simulink model "dvbs2hdlTransmitterCore"  (R2024b)
settings: Solver=FixedStepDiscrete  StartTime=0.0  StopTime=0  RelTol=1e-3
libraries: hdlsllib x105, simulink x41, dspsigops x7, commseqgen3 x5, whdlutilities x5, commhdlcrc x2, dsphdlfiltering2 x1, whdlmod x1
(part 5 of 5)

== system dvbs2hdlTransmitterCore/DVB-S2 Tx/Interleaver/DVB-S2 HDL Interleaver/RAM Address Generator/Read Offset Address/Read Offset Address Signals Generator/FIFO 3 Variables/No HDL/No HDL ==
  wr : Inport
  full : Inport  Port=2
  ncount : Inport  Port=3
  empty : Inport  Port=4
  rd : Inport  Port=5
  Assertion : Assertion  AssertionFailFcn=warning('push on to a full RAM');  StopWhenAssertionFail=off
  Assertion1 : Assertion  AssertionFailFcn=warning('pop from an empty RAM');  StopWhenAssertionFail=off
  Display : Display
  Logical Operator : Logic  Operator=NAND  AllPortsSameDT=off  OutDataTypeStr=boolean
  Logical Operator1 : Logic  Operator=NAND  AllPortsSameDT=off  OutDataTypeStr=boolean
  wires:
  rd/1 -> Logical Operator1/2
  Logical Operator/1 -> Assertion/1
  empty/1 -> Logical Operator1/1
  ncount/1 -> Display/1
  full/1 -> Logical Operator/2
  wr/1 -> Logical Operator/1
  Logical Operator1/1 -> Assertion1/1

== matlab function dvbs2hdlTransmitterCore/DVB-S2 Tx/FEC Encoder/DVB-S2 BCH Encoder/Input controller/Sample Frame type and code rate ==
  data: Enable input; inpFrameLength output; frameTypeIn input; codeRateIdxIn input; inpParityLength output; validateFrameFlag output
function [inpFrameLength,inpParityLength,validateFrameFlag] = sampFramTypeCodeRate(Enable,frameTypeIn,codeRateIdxIn)
%#codegen
%% LUT
inputNFramLenLUT = fi([16008 21408 25728 32208 38688 43040 48408 51648 53840 57472 58192 58192 58192 58192 58192 58192]-1,0,16,0);
inputSFramLenLUT = fi([ 3072  5232  6312  7032  9552 10632 11712 12432 13152 14232 14232 14232 14232 14232 14232 14232]-1,0,14,0);

inpParityNLenLUT = fi([192 192 192 192 192 160 192 192 160 128 128 128 128 128 128 128 ]-1,0,8,0);
inpParitySLenLUT = fi([168 168 168 168 168 168 168 168 168 168 168 168 168 168 168 168]-1,0,8,0);
validateFrameLUT = fi([0 1],0,1,0);

inpFrameLength=cast(0,'like',inputNFramLenLUT);
inpParityLength = cast(0,'like',inpParityNLenLUT);
validateFrameFlag = cast(0,'like',validateFrameLUT);

persistent frameLength;
if isempty(frameLength)
    frameLength=cast(0,'like',inputNFramLenLUT);
end

persistent parityLength;
if isempty(parityLength)
    parityLength=cast(0,'like',inpParityNLenLUT);
end

persistent validateFrame;
if isempty(validateFrame)
    validateFrame=cast(0,'like',validateFrameLUT);
end

%% fetch from inputFramLenLUT
if Enable
    if (~frameTypeIn && codeRateIdxIn <= 10 ) || ( frameTypeIn && codeRateIdxIn <= 9 )
        validateFrameFlag(:) = validateFrameLUT(2);
        validateFrame(:) = validateFrameFlag;
    else
        validateFrameFlag(:) = validateFrameLUT(1);
        validateFrame(:) = validateFrameFlag;
    end
    if frameTypeIn
        inpFrameLength(:)=inputSFramLenLUT(codeRateIdxIn+1);
        frameLength(:)=inputSFramLenLUT(codeRateIdxIn+1);
        inpParityLength(:)=inpParitySLenLUT(codeRateIdxIn+1);
        parityLength(:)=inpParitySLenLUT(codeRateIdxIn+1);
    else
        inpFrameLength(:)=inputNFramLenLUT(codeRateIdxIn+1);
        frameLength(:)=inputNFramLenLUT(codeRateIdxIn+1);
        inpParityLength(:)=inpParityNLenLUT(codeRateIdxIn+1);
        parityLength(:)=inpParityNLenLUT(codeRateIdxIn+1);
    end
else
    inpFrameLength(:)=frameLength;
    inpParityLength(:)=parityLength;
    validateFrameFlag(:) = validateFrame;
end
end

== matlab function dvbs2hdlTransmitterCore/DVB-S2 Tx/FEC Encoder/DVB-S2 BCH Encoder/Input controller/sample bus controller function ==
  data: startIn input; sampledStartIn output; endIn input; validIn input; sampledEndIn output; enbBCHEnc output; reset output
function [sampledStartIn,sampledEndIn,enbBCHEnc,reset] = sampleBusController(startIn,endIn,validIn)
%#codegen
persistent startInTempFlag;
persistent endInFlag;

if isempty(startInTempFlag)
    startInTempFlag =  fi(0,0,1,0);
end
if isempty(endInFlag)
    endInFlag =  fi(0,0,1,0);
end

if endInFlag==1
    startInTempFlag = fi(0,0,1,0);
    endInFlag = fi(0,0,1,0);
end

if startIn==1 && validIn==1 && endIn~=1
    if startInTempFlag==1
        reset = fi(1,0,1,0); %reset
    else
        reset = fi(0,0,1,0);
    end
    sampledStartIn = fi(1,0,1,0); %startSample
    startInTempFlag = fi(1,0,1,0);
else
    sampledStartIn = fi(0,0,1,0);
    reset = fi(0,0,1,0);
end

if startInTempFlag
    enbBCHEnc = fi(1,0,1,0);
else
    enbBCHEnc = fi(0,0,1,0); 
end

if startIn~=1 && endIn==1 && validIn==1 && endInFlag~=1 && startInTempFlag==1
    sampledEndIn = fi(1,0,1,0);
    endInFlag = sampledEndIn;
else
    sampledEndIn = fi(0,0,1,0);
end

== matlab function dvbs2hdlTransmitterCore/DVB-S2 Tx/FEC Encoder/DVB-S2 BCH Encoder/Parity Generation/parity indexing ==
  data: parityVectorInp input; parityScalarOut output; parityScalarValid input; parityIndex input; parityScalarValidOut output; parityLength input
function [parityScalarOut,parityScalarValidOut] = parityIndexing(parityVectorInp,parityScalarValid,parityIndex,parityLength)
%#codegen

parityScalarOut = cast(zeros(1,1),'like',parityScalarValid);
parityScalarValidOut = cast(zeros(1,1),'like',parityScalarValid);

if parityScalarValid 
    parityScalarOut(:) = parityVectorInp(parityIndex+1);
    parityScalarValidOut(:) = parityScalarValid;
else
    parityScalarOut(:) = zeros(1,1);
    parityScalarValidOut(:) = zeros(1,1);
end

== matlab function dvbs2hdlTransmitterCore/DVB-S2 Tx/FEC Encoder/DVB-S2 BCH Encoder/Parity Generation/update parity bits ==
  data: readInpData input; parityBitsVector output size=192; readInpValid input; ParityCalCompFlag input; parityValidVector output; parityValid output; parityLength input; reset input
function [parityBitsVector,parityValidVector,parityValid] = parityBitsUpdater(readInpData,readInpValid,ParityCalCompFlag,parityLength,reset)
%#codegen

persistent writeParData;

parityBuffLen = 192;

if isempty(writeParData) || reset
    writeParData = cast(zeros(parityBuffLen,1),'like',readInpData);
end

parityBits =  cast(zeros(parityBuffLen,1),'like',readInpData);
parityBits(:) =  writeParData;
parityBitsVector = cast(zeros(parityBuffLen,1),'like',readInpData);
parityValidVector = cast(zeros(parityBuffLen,1),'like',readInpData);
parityValid = cast(zeros(1,1),'like',readInpData);
genPoly = cast(zeros(193,1),'like',readInpData);

genPoly192 = cast([1  1   1  0  0  1  1  1  1  0  1  0  1  0  1  0  0  1  0 ...
    0  0  0  0  0  0  1  1  0  0  1  1  0  1  1  1  0  1  1 ...
    1  1  1  0  1  0  0  0  0  1  1  1  1  0  0  0  1  0  1 ...
    1  0  0  0  0  0  0  1  0  0  1  0  0  0  1  0  0  0  1 ...
    0  0  0  0  1  0  1  0  1  1  0  0  0  0  1  1  1  0  1 ...
    1  0  0  0  1  1  0  1  1  0  0  1  1  0  1  0  0  1  1 ...
    1  1  0  0  1  1  0  0  0  0  1  0  1  0  0  0  1  1  1 ...
    0  0  0  1  0  0  0  1  0  1  0  0  0  1  1  1  0  1  0 ...
    0  0  1  0  0  0  0  1  1  1  0  0  0  0  0  1  0  1  1 ...
    1  0  0  0  0  0  1  1  0  0  1  0  0  0  1  1  1  0  0 ...
    1  0  1]','like',readInpData);
genPoly168 = cast([1  0  1  0  0  1  0  1  1  0  1  0  0  0  0  0  1  0  0 ...
    1  1  0  0  0  1  0  0  0  1  0  1  1  1  1  1  0  1  0 ...
    1  1  1  1  1  0  0  1  1  1  1  1  1  1  0  0  0  1  0 ...
    1  0  0  1  0  1  0  1  0  0  1  0  1  1  0  0  0  0  0 ...
    1  0  0  1  1  1  0  0  0  1  0  1  1  1  0  0  0  1  0 ...
    0  1  0  1  1  0  0  1  1  0  1  0  0  0  1  1  0  0  1 ...
    0  0  1  1  0  1  1  0  0  1  0  1  1  0  0  0  0  1  1 ...
    0  0  1  0  1  0  1  0  1  1  1  1  1  0  1  1  0  1  1 ...
    0  1  0  0  0  1  1  0  0  0  0  0  0  0  1  0  1]','like',readInpData);
genPoly160 = cast([1  0  0  0  1  0  0  1  1  0  1  0  0  1  1  0  1  1  0 ...
    1  1  1  0  1  0  0  0  1  1  1  0  1  1  0  0  0  0  0 ...
    0  0  1  1  0  0  0  1  0  0  1  0  0  0  1  0  1  1  1 ...
    1  1  1  0  1  1  1  1  1  0  0  0  0  0  0  1  1  1  0 ...
    1  0  1  0  0  0  0  1  1  1  1  0  0  1  0  1  0  1  1 ...
    0  1  1  1  1  1  0  0  0  1  1  0  0  1  1  0  0  0  1 ...
    0  1  0  1  0  0  0  0  1  1  1  1  1  1  1  0  1  1  0 ...
    1  1  1  0  0  1  1  0  0  0  0  1  0  1  0  1  0  0  0 ...
    0  0  0  0  0  1  1  0  1]','like',readInpData);
genPoly128 = cast([1  1  0  1  0  1  0  0  0  1  1  0  0  1  1  0  1  0  0 ...
    1  1  1  1  1  0  0  1  0  0  0  0  0  1  0  1  0  1  1 ...
    1  0  1  0  1  1  0  1  1  0  0  0  1  1  1  1  1  1  1 ...
    0  0  1  1  0  0  0  1  0  1  1  1  1  0  1  1  1  1  0 ...
    1  0  0  1  1  1  1  0  0  1  0  0  1  0  0  0  1  1  1 ...
    0  1  1  1  1  1  0  1  0  1  0  1  0  0  1  0  0  1  1 ...
    1  0  0  0  0  0  0  0  1  1  1  0  0  0  1]','like',readInpData);
switch parityLength
    case 191
        genPoly(:) = genPoly192;
    case 167
        genPoly(:) = [false(192-168,1); genPoly168 ];
    case 159
        genPoly(:) = [false(192-160,1); genPoly160 ];
    case 127
        genPoly(:) = [false(192-128,1); genPoly128 ];
    otherwise
        genPoly(:) = false(193,1);
end
parityLen192 = length(genPoly192)-1;
if readInpValid
    d = xor(readInpData, parityBits(192));
    for idxPoly = parityLen192 : -1 : 2
        if idxPoly > 192-parityLength
            parityBits(idxPoly) = xor(parityBits(idxPoly-1), (genPoly(idxPoly) & d));
        else
            parityBits(idxPoly) = false;
        end
    end
    parityBits(192-parityLength) = d;
    writeParData(:) = parityBits;
else
    parityBits(:) = writeParData;
end

if ParityCalCompFlag && parityLength == 191
    parityBitsVector(:) = flip(parityBits);
    parityValidVector(:) = ones(parityBuffLen,1);
    parityValid(:) = ones(1,1);
elseif ParityCalCompFlag && parityLength == 167
    parityBitsVector(:) = [flip(parityBits((192-167):192)); false(192-168,1)];
    parityValidVector(:) = [ones(168,1) ; zeros(192-168,1)];
    parityValid(:) = ones(1,1);
elseif ParityCalCompFlag && parityLength == 159
    parityBitsVector(:) = [flip(parityBits((192-159):192)); false(192-160,1)];
    parityValidVector(:) = [ones(160,1) ; zeros(192-160,1)];
    parityValid(:) = ones(1,1);
elseif ParityCalCompFlag && parityLength == 127
    parityBitsVector(:) = [flip(parityBits((192-127):192)); false(192-128,1)];
    parityValidVector(:) = [ones(128,1) ; zeros(192-128,1)];
    parityValid(:) = ones(1,1);
else
    parityBitsVector(:) = zeros(parityBuffLen,1);
    parityValidVector(:) = zeros(parityBuffLen,1);
    parityValid(:) = zeros(1,1);
end

== matlab function dvbs2hdlTransmitterCore/DVB-S2 Tx/FEC Encoder/DVB-S2 LDPC Encoder/Indexing ==
  data: parity output; in_data input; input output; i_index input; par_data input; p_index input
function [parity,input]  = Indexing(in_data,i_index,par_data,p_index)

input = in_data(i_index);
parity = par_data(p_index);

== matlab function dvbs2hdlTransmitterCore/DVB-S2 Tx/FEC Encoder/DVB-S2 LDPC Encoder/Parity RAM/ConvertToMux ==
  data: u1 input; y1 output; u2 input; u3 input; u4 input; y2 output; y3 output; y4 output
function [y1,y2,y3,y4] = fcn(u1,u2,u3,u4)

persistent mux1 mux2 mux3 mux4;
if isempty(mux1)
    mux1 = zeros(90,1)>0;
    mux2 = zeros(90,1)>0;
    mux3 = zeros(90,1)>0;
    mux4 = zeros(90,1)>0;
end

for i =1:90
    mux1(i) = bitget(u1,91-i);
    mux2(i) = bitget(u2,91-i);
    mux3(i) = bitget(u3,91-i);
    mux4(i) = bitget(u4,91-i);
end


y1 = mux1;
y2 = mux2;
y3 = mux3;
y4 = mux4;

== matlab function dvbs2hdlTransmitterCore/DVB-S2 Tx/FEC Encoder/DVB-S2 LDPC Encoder/Parity RAM/ConvertToWord ==
  data: u1 input; y1 output; u2 input; u3 input; u4 input; y2 output; y3 output; y4 output
function [y1,y2,y3,y4] = convertToWord(u1,u2,u3,u4)

y1 = bitconcat(u1);
y2 = bitconcat(u2);
y3 = bitconcat(u3);
y4 = bitconcat(u4);

== matlab function dvbs2hdlTransmitterCore/DVB-S2 Tx/Interleaver/DVB-S2 HDL Interleaver/Discard Out of  Frame samples ==
  data: dataIn input; dataOut output; valid input; validOut output; reset input; fec input
function [dataOut,validOut] = fcn(dataIn,valid,reset,fec)
%#codegen
  
  COUNTMAX_NORMAL = 64800;
  COUNTMAX_SHORT = 16200;

  persistent count dataReg validReg;
  if isempty(count)
      count = fi(COUNTMAX_NORMAL,0,nextpow2(COUNTMAX_NORMAL),0,hdlfimath);
      validReg = false;
      dataReg = cast(0,'like',dataIn);
  end
  
  dataOut = dataReg;
  validOut = validReg;

  if fec
      COUNTMAX = fi(COUNTMAX_SHORT,0,nextpow2(COUNTMAX_NORMAL),0,hdlfimath);
  else
      COUNTMAX = fi(COUNTMAX_NORMAL,0,nextpow2(COUNTMAX_NORMAL),0,hdlfimath);
  end


  if valid && (count < COUNTMAX)
      count(:) = count + 1;
      dataReg = dataIn;
      validReg = valid;
  else
      dataReg(:) = 0;
      validReg = false;
  end
  
  if reset
      count(:) = 0;
  end


end

== matlab function dvbs2hdlTransmitterCore/DVB-S2 Tx/Interleaver/DVB-S2 HDL Interleaver/MATLAB Function ==
  data: valid input; start input; fecFrameIn input; ready output; cnt output; cntval output; modIn input
function [ready,cnt,cntval] = ReadyGenerator(valid,start,fecFrameIn,modIn)
%#codegen

   persistent count countActive countToFrameLength countToFinalValue readyReg;
   if isempty(count)
       count = fi(0,0,nextpow2((64800/2)*8 - 16200),0,hdlfimath);
       countActive = false;
       readyReg = true;
       countToFrameLength = fi(64800,0,nextpow2(64800),0,hdlfimath);
       countToFinalValue = fi((64800/2)*8,0,nextpow2((64800/2)*8),0,hdlfimath);
   end

   ready = readyReg;
   cnt = count;
   cntval = countToFinalValue;

   if start
       if fecFrameIn
           countToFrameLength(:) = 16200;
           switch modIn
               case 0
                   countToFinalValue(:) = (16200/2)*8;
               case 1
                   countToFinalValue(:) = (16200/3)*8;
               case 2
                   countToFinalValue(:) = (16200/4)*8;
               case 3
                   countToFinalValue(:) = (16200/5)*8;
           end
       else
           countToFrameLength(:) = 64800;
           switch modIn
               case 0
                   countToFinalValue(:) = (64800/2)*8;
               case 1
                   countToFinalValue(:) = (64800/3)*8;
               case 2
                   countToFinalValue(:) = (64800/4)*8;
               case 3
                   countToFinalValue(:) = (64800/5)*8;
           end
       end
       countActive = true;
   end

   if countActive 
       if (count < countToFrameLength)
           if valid
               count(:) = count + 1;
           end
           readyReg = true;
       else
           if count == countToFinalValue
               count(:) = 0;
               countActive = false;
               readyReg = true;
           else
               count(:) = count + 1;
               readyReg = false;
           end
       end
   end


end

== matlab function dvbs2hdlTransmitterCore/DVB-S2 Tx/Interleaver/DVB-S2 HDL Interleaver/RAM Address Generator/Read Offset Address/Read Offset Address Signals Generator/Control Logic ==
  data: vMaxR input; chkwrAddrEnd input; vMaxC input; vModCodIs12 input; wrAddr input; curCorROut output; maxRorCOut output; curRorCOut output; modcodIs12Out output; startOut output; endOut output; wrEnb input; modIdx input; readValid output; isInterleave parameter; cnt8 output
function [curCorROut,maxRorCOut,curRorCOut,modcodIs12Out,startOut,endOut,readValid,cnt8] = readAddrCtrl(vMaxR,chkwrAddrEnd,vMaxC,vModCodIs12,wrAddr,wrEnb,modIdx,isInterleave)
%#codegen

    persistent rdEnb rdEnbOld startOutReg;
    persistent curR curC;
    persistent framCnt;
    persistent curCorROutReg maxRorCOutReg curRorCOutReg modcodIs12OutReg;

    persistent wrModIdxReg rdModIdxReg countXOutof8 rdEnbActive;

    if isempty(rdEnb)
        rdEnb           = false;
        rdEnbOld        = false;
        curR            = cast(0,'like',vMaxR);
        curC            = cast(0,'like',vMaxC);
        startOutReg     = false;
        framCnt         = fi(0,0,3,0,hdlfimath);
        
        % XorY => Store X for Interleaver and Y for Deinterleaver
        if isInterleave        
            curCorROutReg   = curC;
            maxRorCOutReg   = vMaxR;
            curRorCOutReg   = curR;
        else
            curCorROutReg   = curR;
            maxRorCOutReg   = vMaxC;
            curRorCOutReg   = curC;
        end
        
        modcodIs12OutReg = vModCodIs12;

        wrModIdxReg        = cast(0,'like',modIdx);
        rdModIdxReg        = cast(0,'like',modIdx);
        countXOutof8     = fi(0,0,3,0);
        rdEnbActive      = false;
    end
    
    curCorROut   = curCorROutReg;
    maxRorCOut   = maxRorCOutReg;
    curRorCOut   = curRorCOutReg;
    modcodIs12Out = modcodIs12OutReg;
    readValid = rdEnbOld;
    startOut  = startOutReg; 
    cnt8 = countXOutof8;
    
    endOut = false;
    if rdEnbOld
        if (isInterleave && (curC == (vMaxC-1))) || (~isInterleave && (curR == (vMaxR-1)))
            if isInterleave
                curC(:) = 0;
            else
                curR(:) = 0;
            end 
            if (~isInterleave && (curC == (vMaxC-1))) || (isInterleave && (curR == (vMaxR-1)))
                if ~isInterleave
                    curC(:) = 0;
                else
                    curR(:) = 0;
                end
                framCnt(:) = framCnt - 1;
                if framCnt == 0
                    rdEnb(:) = false;
                    rdEnbActive = false;
                    if isInterleave
                        curC(:) = 0;
                        curR(:) = 0;
                    end
                end
                endOut = true;
            else
                if isInterleave
                    curR(:) = curR + 1;
                else
                    curC(:) = curC + 1;
                end
            end
        else
            if isInterleave
                curC(:) = curC + 1;
            else
                curR(:) = curR + 1;
            end
        end
    end

    if isInterleave
        if (rdEnbActive && ((curR~=0) || (curC~=0))) || (rdEnbActive && (countXOutof8 == 0))
            if countXOutof8 > fi(rdModIdxReg+1,0,3,0,hdlfimath)
                rdEnb = false;
            else
                rdEnb = true;
            end
        else
            rdEnb = false;
        end
        if countXOutof8 == 7
            countXOutof8(:) = 0;
        else
            countXOutof8(:) = countXOutof8 + 1;
        end
    end
    
    if vModCodIs12 && curC == 0
        curCAdj = cast(2,'like',curC);
    elseif vModCodIs12 && curC == 2
        curCAdj = cast(0,'like',curC);
    else
        curCAdj = curC;
    end
    
    
    if isInterleave
        curCorROutReg    = curCAdj;
        maxRorCOutReg    = vMaxR;
        curRorCOutReg    = curR;
    else
        curCorROutReg    = curR;
        maxRorCOutReg    = vMaxC;
        curRorCOutReg    = curCAdj;
    end
    
    modcodIs12OutReg = vModCodIs12;

    startOutReg = rdEnb && (curR==0) && (curC==0);
    rdEnbOld = rdEnb;
    
    if wrEnb && (wrAddr == chkwrAddrEnd)
        framCnt(:) = framCnt + 1;
        rdEnb(:) = true;

        rdEnbActive = true;
        wrModIdxReg = modIdx;

    end
    if isInterleave && startOutReg
        rdModIdxReg = wrModIdxReg;
    end
    
end

== matlab function dvbs2hdlTransmitterCore/DVB-S2 Tx/MODCOD Source Coder/convertMODCOD ==
  data: modcod input; modIdx output; codIdx output
function [modIdx,codIdx] = convertMODCOD(modcod)
%#codegen

     modIdx = fi(0,0,2,0,hdlfimath);
     codIdx = fi(0,0,4,0,hdlfimath);
     if modcod < 12
         modIdx(:) = 0;
     elseif modcod < 18
         modIdx(:) = 1;
     elseif modcod < 24
         modIdx(:) = 2;
     else
         modIdx(:) = 3;
     end

     switch modcod
         case 1
             codIdx(:) = 0; % 1/4
         case 2
             codIdx(:) =  1; % 1/3
         case 3
             codIdx(:) =  2; % 2/5
         case 4
             codIdx(:) =  3; % 1/2
         case {5,12}
             codIdx(:) =  4; % 3/5
         case {6,13,18}
             codIdx(:) =  5; % 2/3
         case {7,14,19,24}
             codIdx(:) =  6; % 3/4
         case {8,20,25}
             codIdx(:) =  7; % 4/5
         case {9,15,21,26}
             codIdx(:) =  8; % 5/6
         case {10,16,22,27}
             codIdx(:) =  9; % 8/9
         case {11,17,23,28}
             codIdx(:) = 10; % 9/10
         otherwise
             codIdx(:) = 0; % use this as default

     end
end

== matlab function dvbs2hdlTransmitterCore/DVB-S2 Tx/PL Frame Generator/16x ==
  data: trigger input; validOut output
function validOut = monostable(trigger)
%#codegen

   persistent count countActive;
   if isempty(count)
       count = fi(0,0,nextpow2(16 -1),0);
       countActive = false;
   end
   
   validOut = countActive;

   if countActive
       if count == 16-1
           count(:) = 0;
           countActive = false;
       else
           count(:) = count + 1;
       end
   end

   if trigger
       countActive = true;
   end

end

== matlab function dvbs2hdlTransmitterCore/DVB-S2 Tx/PL Frame Generator/Multiplexer/Priority Encoder ==
  data: x1 input; y output; x2 input; x3 input; x4 input
function y = fcn(x1,x2,x3,x4)
%#codegen

  if x4
    y = fi(3,0,2,0);
  elseif x3
      y = fi(2,0,2,0);
  elseif x2
      y = fi(1,0,2,0);
  else
      y = fi(0,0,2,0);
  end

end

== matlab function dvbs2hdlTransmitterCore/DVB-S2 Tx/PL Frame Generator/PL Header Generator/PL Header Bits Generator/Header Bits Packer ==
  data: trigger input; bit7 output; pilotActive input; modcod input; fecframe input; bits1to6 output; start output; valid output
function [bit7,bits1to6,start,valid] = fcn(trigger,pilotActive,modcod,fecframe)
%#codegen
   
   persistent pPilot pModcodFecFrame count countActive;
   if isempty(pPilot)
       pPilot = false;
       pModcodFecFrame = fi(0,0,6,0,hdlfimath);
       count = fi(0,0,3,0,hdlfimath);
       countActive = false;
   end

   bit7 = pPilot;
   bits1to6 = bitget(pModcodFecFrame,5-count+1);
   start = (count == 0) && countActive;
   valid = countActive;

   if countActive
       if count == 5
           count(:) = 0;
           countActive = false;
       else
           count(:) = count + 1;
       end
   end

   if trigger
       pPilot = pilotActive;
       pModcodFecFrame = bitconcat(fi(modcod,hdlfimath),fi(fecframe,hdlfimath));
       countActive = true;
   end

end

== matlab function dvbs2hdlTransmitterCore/DVB-S2 Tx/PL Frame Generator/PL Header Generator/PL Header Bits Generator/PLSC Generator/Serialize on trigger ==
  data: data input; dataOut output; validOut output; startOut output; trigger input
function [dataOut,validOut,startOut] = fcn(data,trigger)
%#codegen

    persistent count countActive;
    if isempty(count)
        count               = fi(0,0,5,0,hdlfimath);
        countActive         = false;
    end
    
    dataOut                 = data(fi(count + 1,0,6,0));
    startOut                = (count == 0) && countActive;
    validOut                = countActive;

    if countActive
        if count == 31
            count(:)        = 0;
            countActive(:)  = 0;
        else
            count(:)        = count + 1;
        end
    end

    if trigger
        countActive         = true;
    end

end

== matlab function dvbs2hdlTransmitterCore/DVB-S2 Tx/PL Frame Generator/PL Header Generator/PL Header Bits Generator/SOF Generator/SOF Sequence LUT Address Generator ==
  data: trigger input; LUTAddr output; valid output
function [LUTAddr,valid] = fcn(trigger)
%#codegen

   persistent count countActive;
   if isempty(count)
       count             = fi(0,0,nextpow2(25),0,hdlfimath);
       countActive       = false;
   end

   LUTAddr               = count;
   valid                 = countActive;

   if countActive
       if count == 25
           count(:)      = 0;
           countActive   = false;
       else
           count(:)      = count + 1;
       end
   end

   if trigger
       countActive       = true;
   end

end

== matlab function dvbs2hdlTransmitterCore/DVB-S2 Tx/PL Frame Generator/RAM FIFO/PL Data FIFO/Dummy Frame Generator/Dummy Frame Header LUT Address Generator ==
  data: countOut output; validm2 output; nextFrameReady input; valid output; EOF input
function [countOut,validm2,valid] = fcn(nextFrameReady,EOF)
%#codegen
  
  dummyFrameLength = 90 + 36*90;
  persistent count countActive;
  if isempty(count)
      count = fi(0,0,nextpow2(dummyFrameLength - 1),0,hdlfimath);
      countActive = false;
  end

  if ~countActive && EOF && ~nextFrameReady
      countActive = true;
  end

  valid = countActive;
  validm2 = countActive && (count<=dummyFrameLength-3);
  countOut = count;
  
  if countActive
      if count == dummyFrameLength-1
          count(:) = 0;
          countActive = false;
      else
          count(:) = count + 1;
      end
  end

end

== matlab function dvbs2hdlTransmitterCore/DVB-S2 Tx/PL Frame Generator/RAM FIFO/PL Data FIFO/Frame Length FIFO/No HDL/RAM status ==
  data: full output; ncount output; wr input; empty output; rd input
function [full,ncount,empty] = fcn(wr,rd)
%#codegen
     
    WL = 4;
    persistent count;
    if isempty(count)
        count = fi(0,0,WL+1,0,hdlfimath);
    end

    empty = (count == 0);
    full = (count > 2^WL-1);
    ncount = count;

    if wr
        count(:) = count + 1;
    end
    if rd
        count(:) = count - 1;
    end

end

== matlab function dvbs2hdlTransmitterCore/DVB-S2 Tx/PL Frame Generator/RAM FIFO/PL Data FIFO/In Frame Count ==
  data: countOut output; enb input; endOut output; countToValue input
function [countOut,endOut] = counter(enb,countToValue)
%#codegen

   persistent count;
   if isempty(count)
       count = cast(0,'like',countToValue);
   end
   
   countOut = count;
   if countToValue == 0
       endOut = false;
   else
       endOut = (count == countToValue-1) && enb;
   end

   if enb
       if (count ~= 0) && (count == countToValue-1)
           count(:) = 0;
       else
           count(:) = count + 1;
       end
   end

end

== matlab function dvbs2hdlTransmitterCore/DVB-S2 Tx/PL Frame Generator/RAM FIFO/PL Data FIFO/Out Frame Count ==
  data: startOutFrame output; endOutFrame output; endOutFramem2 output; endOut16Slots output; validOut output; endOfPLHeader input; endOfPilotBlk input; frameLength input
function [startOutFrame,endOutFrame,endOutFramem2,endOut16Slots,validOut] = counter(endOfPLHeader,endOfPilotBlk,frameLength)
%#codegen

   LENGTH = 90*16;
   persistent slotCount countActive slotEnd frameCount;
   if isempty(slotCount)
       slotCount = fi(0,0,nextpow2(LENGTH -1),0);
       countActive = false;
       slotEnd = false;
       frameCount = cast(0,'like',frameLength);
   end
   
   endOut16Slots = slotEnd;
   validOut = countActive;
   endOutFrame = countActive && (frameCount == frameLength-1);
   endOutFramem2 = countActive && (frameCount == frameLength-1-2);
   startOutFrame = countActive && (frameCount == 0);

   if countActive && (frameCount == frameLength-1)
       slotCount(:) = 0;
       countActive = false;
       slotEnd = false;
       frameCount(:) = 0;
   else
       if countActive
           frameCount(:) = frameCount + 1;
           if slotCount == LENGTH-1
               slotCount(:) = 0;
               countActive = false;
           else
               slotCount(:) = slotCount + 1;
           end
           if slotCount == LENGTH-1
               slotEnd = true;
           else
               slotEnd = false;
           end
       else
           slotEnd = false;
       end

       if (endOfPLHeader && (frameCount == 0)) || (endOfPilotBlk && (frameCount ~= 0))
           countActive = true;
       end
   end

end

== matlab function dvbs2hdlTransmitterCore/DVB-S2 Tx/BB Frame Generator/BB Header and Data CRC Generator/BB Header Generator/BB Header Packetizer ==
  data: startIn input; TSorGS input; dataOut output; startOut output; endOut output; validOut output; DFL input; UPL input; SYNC input; countOut output
function [dataOut,startOut,endOut,validOut,countOut] = BBHeaderCount(startIn,TSorGS,DFL,UPL,SYNC)
%#codegen

persistent count dataReg startReg endReg validReg;
   if isempty(count)
       count = fi(72,0,nextpow2(80),0,hdlfimath);
       dataReg = false;
       startReg = false;
       endReg = false;
       validReg = false;
   end

   dataOut = dataReg;
   startOut = startReg;
   endOut = endReg;
   validOut = validReg;
   countOut = count;
   
   dataReg = false;
   validReg = false;
   startReg = false;
   endReg = false;
   
   if startIn
       count(:) = 0;
   end
   
       if count < 72
           validReg = true;
           if count == 0
               dataReg = logical(bitget(TSorGS,2));       % MSB of TS/GS
               startReg = true;                           % start of header
           elseif count == 1
               dataReg = logical(bitget(TSorGS,1));       % LSB of TS/GS
           elseif (count == 2) || (count == 3)
               dataReg = true;                            % SIS/MIS, CCM/ACM
%            elseif (count >= 4) && (count <= 15)           % ISSYI, NPD, RO, MATTYPE-2
           elseif (count >= 16) && (count <= 31)
               dataReg = logical(bitget(UPL,uint8(32-count)));   % UPL
           elseif (count >= 32) && (count <= 47) % DFL
               dataReg = logical(bitget(DFL,uint8(48-count)));   % DFL
           elseif (count >= 48) && (count <= 55)          % SYNC
               dataReg = logical(bitget(SYNC,uint8(56-count)));
%            elseif (count >= 56) && (count <= 71)          % SYNCD
           elseif count == 71
               endReg = true;                             % end of header
           end
           count(:) = count + 1;
       else
           validReg = false;
       end
   

end

== matlab function dvbs2hdlTransmitterCore/DVB-S2 Tx/PL Frame Generator/RAM FIFO/PL Data FIFO/No HDL/RAM status ==
  data: full output; ncount output; wr input; empty output; rd input
function [full,ncount,empty] = fcn(wr,rd)
%#codegen
     
    WL = 16;
    persistent count;
    if isempty(count)
        count = fi(0,0,WL+1,0,hdlfimath);
    end

    empty = (count == 0);
    full = (count > 2^WL-1);
    ncount = count;

    if wr
        count(:) = count + 1;
    end
    if rd
        count(:) = count - 1;
    end

end

== matlab function dvbs2hdlTransmitterCore/DVB-S2 Tx/PL Frame Generator/RAM FIFO/PL Header FIFO/90x ==
  data: validOut output; startOut output; endOut output; trigger input; endOutm1 output
function [validOut,startOut,endOut,endOutm1] = monostable(trigger)
%#codegen
   
   LENGTH = 90;
   persistent count countActive;
   if isempty(count)
       count = fi(0,0,nextpow2(LENGTH-1),0);
       countActive = false;
   end
   
   validOut = countActive;
   endOut = (count == LENGTH-1) && countActive;
   endOutm1 = (count == LENGTH-2) && countActive;
   startOut = (count == 0) && countActive;

   if countActive
       if count == LENGTH-1
           count(:) = 0;
           countActive = false;
       else
           count(:) = count + 1;
       end
   end

   if trigger
       countActive = true;
   end

end

== matlab function dvbs2hdlTransmitterCore/DVB-S2 Tx/PL Frame Generator/RAM FIFO/PL Header FIFO/No HDL/RAM status ==
  data: full output; ncount output; wr input; empty output; rd input
function [full,ncount,empty] = fcn(wr,rd)
%#codegen
     
    WL = nextpow2(450);
    persistent count;
    if isempty(count)
        count = fi(0,0,WL+1,0,hdlfimath);
    end

    empty = (count == 0);
    full = (count > 2^WL-1);
    ncount = count;

    if wr
        count(:) = count + 1;
    end
    if rd
        count(:) = count - 1;
    end

end

== matlab function dvbs2hdlTransmitterCore/DVB-S2 Tx/PL Frame Generator/RAM FIFO/Pilot Generator/Pilot Block Length Valid Generator ==
  data: endOut output; endOutm1 output; trigger input; validOut output
function [endOut,endOutm1,validOut] = monostable(trigger)
%#codegen

   LENGTH = 36;
   persistent count countActive countEnd countEndm1;
   if isempty(count)
       count = fi(0,0,nextpow2(LENGTH -1),0);
       countActive = false;
       countEnd = false;
       countEndm1 = false;
   end
   
   endOut = countEnd;
   validOut = countActive;
   endOutm1 = countEndm1;

   if countActive
       if count == LENGTH-1
           count(:) = 0;
           countActive = false;
       else
           count(:) = count + 1;
       end
       if count == LENGTH-2
           countEndm1 = true;
       else
           countEndm1 = false;
       end
       if count == LENGTH-1
           countEnd = true;
       else
           countEnd = false;
       end
   else
       countEnd = false;
       countEndm1 = false;
   end


   if trigger
       countActive = true;
   end

end

== matlab function dvbs2hdlTransmitterCore/DVB-S2 Tx/PL Frame Generator/Subsystem/8x ==
  data: startIn input; endIn input; startOut output; validOut output
function [startOut,validOut] = monostable(startIn,endIn)
%#codegen
   
   LENGTH = 8;
   persistent count countActive isEndReceived startReg validReg;
   if isempty(count)
       count = fi(0,0,nextpow2(LENGTH-1),0);
       countActive = false;
       isEndReceived = false;
       startReg = false;
       validReg = false;
   end

   startOut = startReg;
   validOut = validReg;

   if startIn
       countActive = true;
       startReg = true;
   end

   validReg = countActive;
   

   if endIn
       isEndReceived = true;
   end

   if countActive
       if count == LENGTH-1
           count(:) = 0;
           startReg = false;
           if isEndReceived
               isEndReceived = false;
               countActive = false;
           end
       else
           count(:) = count + 1;
       end
           
   end

end

== matlab function dvbs2hdlTransmitterCore/DVB-S2 Tx/FEC Encoder/DVB-S2 LDPC Encoder/ParityController ==
  data: ird_addr output; pwr_addr output; pwr_enb output; prd_addr output; endEnc input; paraddr input; encenable input; inpLen input; parLen input; qfactor input; noofcol input; reset input; starto output; endo output; valido output; par_ind output; i_index output; p_index output; framevalid input
function [ird_addr,pwr_addr,pwr_enb,prd_addr,starto,endo,valido,par_ind,...
    i_index,p_index] = ParityController(endEnc,paraddr,encenable,...
    inpLen,parLen,qfactor,noofcol,reset,framevalid)

persistent validO prdAddr pwrAddr pwrEnb pwrEnbReg ...
    irdAddr prdEnb endValid startO icountZ inCount ...
    parCount pcountZ;
if isempty(validO)
    validO = false;
    prdAddr = uint8(1);
    pwrAddr = uint8(0);
    irdAddr = uint8(1);
    pwrEnb = false;
    pwrEnbReg = false;
    prdEnb = false;
    endValid = false;
    startO = false;
    icountZ = fi(1,0,9,0,hdlfimath);
    pcountZ = fi(1,0,9,0,hdlfimath);
    inCount = fi(0,0,16,0,hdlfimath);
    parCount = fi(0,0,16,0,hdlfimath);
end

ird_addr = irdAddr;
pwr_addr = pwrAddr;
prd_addr = prdAddr;
pwr_enb =  pwrEnbReg;
starto = startO;
par_ind = prdEnb;

i_index = icountZ;
p_index = pcountZ;

% Control signals
startO = endEnc;
endo = endValid;
valido = validO && ~endValid;

pwrEnbReg(:) = pwrEnb;

if reset
    prdAddr(:) = 1;
    pwrAddr(:) = 0;
    pwrEnb(:) = false;
    prdEnb(:) = false;
    endValid(:) = false;
    irdAddr(:) = 1;
    icountZ(:) = 1;
    pcountZ(:) = 1;
    inCount(:) = 0;
    parCount(:) = 0;
else
    if validO
        pwrEnb(:) = false;
        pwrAddr(:) = 0;

        if ~prdEnb
            if icountZ == fi(360,0,9,0,hdlfimath)
                if ~(irdAddr == noofcol)
                    irdAddr(:) = irdAddr + 1;
                end
                icountZ(:) = 1;
            else
                icountZ(:) = icountZ + 1;
            end
        end

        if inCount == inpLen
            prdEnb(:) = true;
        else
            inCount(:) = inCount + 1;
        end

        if prdEnb
            if parCount == parLen
                prdEnb(:) = false;
                endValid(:) = true;
            else
                parCount(:) = parCount + 1;
                if prdAddr == fi(qfactor,0,9,0,hdlfimath)
                    prdAddr(:) = 1;
                    if pcountZ == fi(360,0,9,0,hdlfimath)
                        pcountZ(:) = 1;
                    else
                        pcountZ(:) = pcountZ + 1;
                    end
                else
                    prdAddr(:) = prdAddr + 1;
                end
            end
        else
            prdAddr(:) = 1;
            endValid(:) = false;
        end
    else
        if framevalid
            pwrEnb(:) = true;
            if pwrAddr == uint8(255)
                pwrAddr(:) = 1;
            else
                pwrAddr(:) = pwrAddr+1;
            end
        else
            if encenable
                pwrEnb(:) = true;
            else
                pwrEnb(:) = false;
            end
            pwrAddr(:) = prdAddr;
        end
        prdAddr(:) = paraddr;
        prdEnb(:) = false;
        endValid(:) = false;
    end
end

if reset || endValid
    validO(:) = false;
elseif endEnc
    validO(:) = true;
end

== matlab function dvbs2hdlTransmitterCore/DVB-S2 Tx/FEC Encoder/DVB-S2 LDPC Encoder/inputController ==
  data: reset output; datai input; iwr_data output size=360; iwr_addr output; starti input; endi input; validi input; fecframe input; coderate input; iwr_enb output size=360; ird_addr output; encenable output; addridx output; rdenable input; encend input; framevalid output; noofcol input
function [reset,iwr_data, iwr_addr,iwr_enb,ird_addr,encenable,addridx,framevalid] = ...
    inputController(datai,starti,endi,validi,fecframe,coderate,rdenable,encend,noofcol)
%#codegen

persistent fecFrame codeRate dataReg endReg validReg frameValid  frameValidReg...
           iwrData iwrAddr iwrEnb irdAddr idxCount wrCount encEnb disValid;
if isempty(dataReg)
    fecFrame = fi(0,0,1,0);
    codeRate = fi(0,0,4,0);
    dataReg = cast(0,'like',datai);
    endReg = false;
    validReg = false;
    frameValid = false;
    frameValidReg = false;
    iwrData = cast(zeros(360,1),'like',datai);
    iwrAddr = fi(0,0,8,0,hdlfimath);
    iwrEnb  = zeros(360,1)>0;
    irdAddr = fi(0,0,8,0,hdlfimath);
    idxCount = fi(1,0,9,0,hdlfimath);
    wrCount = fi(1,0,8,0,hdlfimath);
    encEnb = false;
    disValid = false;
end

% outputs
iwr_data = iwrData;
iwr_addr = iwrAddr;
iwr_enb = iwrEnb;
ird_addr = irdAddr;
encenable = disValid;

%% reset signal
reset = starti && validi;

%% Sample fecFrame and codeRate - Calculate input,parity length and address index.
if reset
    fecFrame(:) = fecframe;
    codeRate(:) = coderate;
end

addridx = fi(bitconcat(fecFrame,codeRate),0,5,0);

%% Reading data
if reset
    irdAddr(:) = 1;
else
    if rdenable
        if irdAddr == cast(noofcol,'like',irdAddr)
            irdAddr(:) = 1;
        else
            irdAddr(:) = irdAddr + 1;
        end
    end
end

%% Writing and Reading data into Input Bits RAM
if reset
    iwrData(:) = zeros(360,1);
    iwrAddr(:) = 0;
    iwrEnb(:) = zeros(360,1);
    idxCount(:) = 1;
    wrCount(:) = 1;
else
    if frameValid && validReg
        for idx = 1:360
            if idxCount == fi(idx,0,9,0)
                iwrEnb(idx) = true;
                iwrData(idx) = dataReg;
            else
                iwrEnb(idx) = false;
                iwrData(idx) = 0;
            end
        end
        iwrAddr(:) = wrCount;
        if idxCount == fi(360,0,9,0)
            idxCount(:) = 1;
            wrCount(:) = wrCount + 1;
        else
            idxCount(:) = idxCount + 1;
        end
    else
        iwrData(:) = 0;
        iwrEnb(:)  = false;
    end
end

if reset
    frameValid(:) = true;
    encEnb(:) = false;
elseif endReg && validReg
    frameValid(:) = false;
    encEnb(:) = true;
elseif encend
    encEnb(:) = false;
end

if reset
    frameValidReg(:) = true;
elseif endi && validi
    frameValidReg(:) = false;
end

if encEnb
    disValid(:) = ~disValid;
else
    disValid(:) = false;
end

framevalid = frameValidReg;

dataReg(:) = datai;
endReg(:) = endi;
validReg(:) = validi;

== matlab function dvbs2hdlTransmitterCore/DVB-S2 Tx/Interleaver/DVB-S2 HDL Interleaver/RAM Address Generator/Read Offset Address/Read Offset Address Signals Generator/FIFO 3 Variables/No HDL/RAM status ==
  data: full output; ncount output; wr input; empty output; rd input
function [full,ncount,empty] = fcn(wr,rd)
%#codegen
     
    WL = 3;
    persistent count;
    if isempty(count)
        count = fi(0,0,WL+1,0,hdlfimath);
    end

    empty = (count == 0);
    full = (count > 2^WL-1);
    ncount = count;

    if wr
        count(:) = count + 1;
    end
    if rd
        count(:) = count - 1;
    end

end

== matlab function dvbs2hdlTransmitterCore/DVB-S2 Tx/BB Frame Generator/BB Header and Data CRC Generator/Data Field Generator/Packetized Streams/Discard SYNC ==
  data: dataIn input; dataOut output; startIn input; endIn input; validIn input; startOut output; endOut output; validOut output
function [dataOut,startOut,endOut,validOut] = discardSYNC(dataIn,startIn,endIn,validIn)
%#codegen


persistent count dataReg validReg startReg endReg;
    if isempty(count)
        count = fi(0,0,4,0,hdlfimath);
        dataReg = cast(0,'like',dataIn);
        validReg = false;
        startReg = false;
        endReg = false;
    end

    dataOut = dataReg;
    validOut = validReg;
    startOut = startReg;
    endOut = endReg;

    if startIn
        count(:) = 0;
    end
 
    if validIn
        if (count < 8)
            startReg = false;
            validReg = false;
        elseif count == 8
            startReg = true;
            validReg = true;
        else
            startReg = false;
            validReg = true;
        end
        if count < 9
            count(:) = count + 1;
        end
    else
        validReg = false;
        startReg = false;
    end
    if validReg
        dataReg = dataIn;
        endReg = endIn;
    else
        dataReg(:) = 0;
        endReg = false;
    end

end

== matlab function dvbs2hdlTransmitterCore/DVB-S2 Tx/BB Frame Generator/BB Header and Data CRC Generator/Data Field Generator/Packetized Streams/MATLAB Function ==
  data: pktEndIn input; frameEndOut output; frameEndIn input
function frameEndOut = fcn(pktEndIn,frameEndIn)
%#codegen

    persistent frameEnded;
    if isempty(frameEnded)
        frameEnded = false;
    end

    if frameEndIn
        frameEnded = true;
    end

    if pktEndIn && frameEnded
        frameEndOut = true;
        frameEnded = false;
    else
        frameEndOut = false;
    end


end

== matlab function dvbs2hdlTransmitterCore/DVB-S2 Tx/BB Frame Generator/BB Header and Data CRC Generator/MATLAB Function ==
  data: validIn input; startIn input; endIn input; validAppend output; DFL input; endAppend output
function [validAppend,endAppend] = DFLLengthCounter(validIn,startIn,endIn,DFL)
%#codegen
   
   MAX_DFL = 58192-80; 
   persistent countDFL isEndReceived;
   if isempty(countDFL)
       countDFL = fi(0,0,nextpow2(MAX_DFL),0,hdlfimath);
       isEndReceived = false;
   end
   
   if startIn
       countDFL(:) = 0;
   end

   if isEndReceived
       validAppend = true;
       countDFL(:) = countDFL + 1;
   elseif validIn
       validAppend = false;
       countDFL(:) = countDFL + 1;
   else
       validAppend = false;
   end
   
   if countDFL > DFL
       validAppend = false;
   end
   if DFL ~= 0
       if countDFL >= DFL
           endAppend = isEndReceived;
           isEndReceived = false;
       else
           endAppend = false;
       end
   else
       endAppend = false;
   end

   if endIn
       isEndReceived = true;
   end
end

== matlab function dvbs2hdlTransmitterCore/DVB-S2 Tx/BB Frame Generator/BB Header and Data CRC Generator/No HDL/MATLAB Function1 ==
  data: u input; y output
function y = monostable(u)
%#codegen

   persistent count countActive;
   if isempty(count)
       count = fi(0,0,nextpow2(80),0,hdlfimath);
       countActive = false;
   end

   y = countActive;
    
   if count == 79
       countActive = false;
       count(:) = 0;
   end
   if countActive
       count(:) = count + 1;
   end
   if u 
       countActive = true;
   end

end

== matlab function dvbs2hdlTransmitterCore/DVB-S2 Tx/BB Frame Generator/Data Store FIFO/MATLAB Function ==
  data: wr input; startIn input; validOut output; DFL input; endOut output
function [validOut,endOut] = DFLLengthCounter(wr,startIn,DFL)
%#codegen
   
   WL = 7;
   persistent countDFL countActive countSamplesInRAM;
   if isempty(countDFL)
       countDFL = cast(0,'like',DFL);
       countActive = false;
       countSamplesInRAM = fi(0,0,WL+1,0,hdlfimath);

   end

   empty = (countSamplesInRAM == 0);
   enb = ~empty;
   % cntActive = countActive;
   % cnt = countDFL;

   validOut = countActive && enb;
   endOut = countActive && (countDFL == DFL);


   if (DFL ~= 0) && (countDFL == DFL) && enb
       countActive = false;
   end

   if startIn
       countDFL(:) = 0;
       countActive = true;
   end

   if countActive && enb
       countDFL(:) = countDFL + 1;
   end



   if wr
       countSamplesInRAM(:) = countSamplesInRAM + 1;
   end
   if validOut % rd
       countSamplesInRAM(:) = countSamplesInRAM - 1;
   end



end

== matlab function dvbs2hdlTransmitterCore/DVB-S2 Tx/BB Frame Generator/Data Store FIFO/No HDL/RAM status ==
  data: full output; ncount output; wr input; empty output; rd input
function [full,ncount,empty] = fcn(wr,rd)
%#codegen
     
    WL = 7;
    persistent count;
    if isempty(count)
        count = fi(0,0,WL+1,0,hdlfimath);
    end

    empty = (count == 0);
    full = (count > 2^WL-1);
    ncount = count;

    if wr
        count(:) = count + 1;
    end
    if rd
        count(:) = count - 1;
    end

end
